simulink model "case4"  (R2024b)
settings: Solver=FixedStepAuto  StartTime=0  StopTime=1  FixedStep=1e-7  RelTol=1e-3
values from neighbouring files (symbols this model uses):
  SG_D_1_D = 0.01056    [IEEE9_case_parameters.m]    (also in case1_parameters.m; case2_parameters.m; case3_parameters.m; case4_parameters.m)
  SG_D_1_EnableSaturation = 0    [IEEE9_case_parameters.m]    (also in case1_parameters.m; case2_parameters.m; case3_parameters.m; case4_parameters.m)
  SG_D_1_f0 = 60    [IEEE9_case_parameters.m]    (also in case1_parameters.m; case2_parameters.m; case3_parameters.m; case4_parameters.m)
  SG_D_1_H = 7.5    [IEEE9_case_parameters.m]    (also in case1_parameters.m; case2_parameters.m; case3_parameters.m; case4_parameters.m)
  SG_D_1_K_A = 20    [IEEE9_case_parameters.m]    (also in case1_parameters.m; case2_parameters.m; case3_parameters.m; case4_parameters.m)
  SG_D_1_K_E = 1.000000e+1    (= 10)    [IEEE9_case_parameters.m]    (also in case1_parameters.m; case2_parameters.m; case3_parameters.m; case4_parameters.m)
  SG_D_1_K_F = 2.363    [IEEE9_case_parameters.m]    (also in case1_parameters.m; case2_parameters.m; case3_parameters.m; case4_parameters.m)
  SG_D_1_K_s = 0.5    [IEEE9_case_parameters.m]    (also in case1_parameters.m = 5; case2_parameters.m = 5; case3_parameters.m = 5; case4_parameters.m = 5)
  SG_D_1_R_a = 0.001088    [IEEE9_case_parameters.m]    (also in case1_parameters.m; case2_parameters.m; case3_parameters.m; case4_parameters.m)
  SG_D_1_S_A = 1    [IEEE9_case_parameters.m]    (also in case1_parameters.m; case2_parameters.m; case3_parameters.m; case4_parameters.m)
  SG_D_1_S_B = 0.103    [IEEE9_case_parameters.m]    (also in case1_parameters.m; case2_parameters.m; case3_parameters.m; case4_parameters.m)
  SG_D_1_S_N = 10.659857    [IEEE9_case_parameters.m]    (also in case1_parameters.m; case2_parameters.m; case3_parameters.m; case4_parameters.m)
  SG_D_1_SpeedPara = 200    [IEEE9_case_parameters.m]    (also in case1_parameters.m; case2_parameters.m; case3_parameters.m; case4_parameters.m)
  SG_D_1_T_0 = 0.720173    [IEEE9_case_parameters.m]    (also in case1_parameters.m = 0.755522; case2_parameters.m = 0.808931; case3_parameters.m = 0.869402; case4_parameters.m = 0.729316)
  SG_D_1_T_1 = 0.3    [IEEE9_case_parameters.m]    (also in case1_parameters.m; case2_parameters.m; case3_parameters.m; case4_parameters.m)
  SG_D_1_T_2 = 0.05    [IEEE9_case_parameters.m]    (also in case1_parameters.m; case2_parameters.m; case3_parameters.m; case4_parameters.m)
  SG_D_1_T_3 = 0.02    [IEEE9_case_parameters.m]    (also in case1_parameters.m; case2_parameters.m; case3_parameters.m; case4_parameters.m)
  SG_D_1_T_4 = 0.005    [IEEE9_case_parameters.m]    (also in case1_parameters.m; case2_parameters.m; case3_parameters.m; case4_parameters.m)
  SG_D_1_T_A = 0.02    [IEEE9_case_parameters.m]    (also in case1_parameters.m; case2_parameters.m; case3_parameters.m; case4_parameters.m)
  SG_D_1_T_dd = 8.000000e+0    (= 8)    [IEEE9_case_parameters.m]    (also in case1_parameters.m; case2_parameters.m; case3_parameters.m; case4_parameters.m)
  SG_D_1_T_ddd = 0.04    [IEEE9_case_parameters.m]    (also in case1_parameters.m; case2_parameters.m; case3_parameters.m; case4_parameters.m)
  SG_D_1_T_E = 0.314    [IEEE9_case_parameters.m]    (also in case1_parameters.m; case2_parameters.m; case3_parameters.m; case4_parameters.m)
  SG_D_1_T_F = 0.35    [IEEE9_case_parameters.m]    (also in case1_parameters.m; case2_parameters.m; case3_parameters.m; case4_parameters.m)
  SG_D_1_T_qd = 0.8    [IEEE9_case_parameters.m]    (also in case1_parameters.m; case2_parameters.m; case3_parameters.m; case4_parameters.m)
  SG_D_1_T_qdd = 0.02    [IEEE9_case_parameters.m]    (also in case1_parameters.m; case2_parameters.m; case3_parameters.m; case4_parameters.m)
  SG_D_1_T_speed = 0.1    [IEEE9_case_parameters.m]    (also in case1_parameters.m = 200; case2_parameters.m = 200; case3_parameters.m = 200; case4_parameters.m = 200)
  SG_D_1_T_w = 0.5    [IEEE9_case_parameters.m]    (also in case1_parameters.m; case2_parameters.m; case3_parameters.m; case4_parameters.m)
  SG_D_1_V_ref = 1.990276    [IEEE9_case_parameters.m]    (also in case1_parameters.m = 2.042296; case2_parameters.m = 2.051388; case3_parameters.m = 2.089584; case4_parameters.m = 2.01845)
  SG_D_1_w_ref = 376.991118    [IEEE9_case_parameters.m]    (also in case1_parameters.m; case2_parameters.m; case3_parameters.m; case4_parameters.m)
  SG_D_1_wb = 6.000000e+1    (= 60)    [IEEE9_case_parameters.m]    (also in case1_parameters.m; case2_parameters.m; case3_parameters.m; case4_parameters.m)
  SG_D_1_x_d = 1.9    [IEEE9_case_parameters.m]    (also in case1_parameters.m; case2_parameters.m; case3_parameters.m; case4_parameters.m)
  SG_D_1_x_dd = 0.302    [IEEE9_case_parameters.m]    (also in case1_parameters.m; case2_parameters.m; case3_parameters.m; case4_parameters.m)
  SG_D_1_x_ddd = 0.204    [IEEE9_case_parameters.m]    (also in case1_parameters.m; case2_parameters.m; case3_parameters.m; case4_parameters.m)
  SG_D_1_x_l = 0.05    [IEEE9_case_parameters.m]    (also in case1_parameters.m; case2_parameters.m; case3_parameters.m; case4_parameters.m)
  SG_D_1_x_q = 1.3    [IEEE9_case_parameters.m]    (also in case1_parameters.m; case2_parameters.m; case3_parameters.m; case4_parameters.m)
  SG_D_1_x_qd = 0.5    [IEEE9_case_parameters.m]    (also in case1_parameters.m; case2_parameters.m; case3_parameters.m; case4_parameters.m)
  SG_D_1_x_qdd = 0.3    [IEEE9_case_parameters.m]    (also in case1_parameters.m; case2_parameters.m; case3_parameters.m; case4_parameters.m)
  SG_D_2_D = 0.02    [IEEE9_case_parameters.m]    (also in case1_parameters.m; case2_parameters.m; case3_parameters.m; case4_parameters.m)
  SG_D_2_EnableSaturation = 0    [IEEE9_case_parameters.m]    (also in case1_parameters.m; case2_parameters.m; case3_parameters.m; case4_parameters.m)
  SG_D_2_f0 = 60    [IEEE9_case_parameters.m]    (also in case1_parameters.m; case2_parameters.m; case3_parameters.m; case4_parameters.m)
  SG_D_2_H = 8.000000e+0    (= 8)    [IEEE9_case_parameters.m]    (also in case1_parameters.m; case2_parameters.m; case3_parameters.m; case4_parameters.m)
  SG_D_2_K_A = 20    [IEEE9_case_parameters.m]    (also in case1_parameters.m; case2_parameters.m; case3_parameters.m; case4_parameters.m)
  SG_D_2_K_E = 1.000000e+1    (= 10)    [IEEE9_case_parameters.m]    (also in case1_parameters.m; case2_parameters.m; case3_parameters.m; case4_parameters.m)
  SG_D_2_K_F = 2.363    [IEEE9_case_parameters.m]    (also in case1_parameters.m; case2_parameters.m; case3_parameters.m; case4_parameters.m)
  SG_D_2_K_s = 0.5    [IEEE9_case_parameters.m]    (also in case1_parameters.m = 4; case2_parameters.m = 4; case3_parameters.m = 4; case4_parameters.m = 4)
  SG_D_2_R_a = 0.001088    [IEEE9_case_parameters.m]    (also in case1_parameters.m; case2_parameters.m; case3_parameters.m; case4_parameters.m)
  SG_D_2_S_A = 1    [IEEE9_case_parameters.m]    (also in case1_parameters.m; case2_parameters.m; case3_parameters.m; case4_parameters.m)
  SG_D_2_S_B = 0.103    [IEEE9_case_parameters.m]    (also in case1_parameters.m; case2_parameters.m; case3_parameters.m; case4_parameters.m)
  SG_D_2_S_N = 10.659857    [IEEE9_case_parameters.m]    (also in case1_parameters.m; case2_parameters.m; case3_parameters.m; case4_parameters.m)
  SG_D_2_SpeedPara = 200    [IEEE9_case_parameters.m]    (also in case1_parameters.m; case2_parameters.m; case3_parameters.m; case4_parameters.m)
  SG_D_2_T_0 = 1.632913    [IEEE9_case_parameters.m]    (also in case1_parameters.m = 1.632925; case2_parameters.m = 1.632915; case3_parameters.m = 1.632914; case4_parameters.m = 1.632927)
  SG_D_2_T_1 = 0.2    [IEEE9_case_parameters.m]    (also in case1_parameters.m; case2_parameters.m; case3_parameters.m; case4_parameters.m)
  SG_D_2_T_2 = 0.05    [IEEE9_case_parameters.m]    (also in case1_parameters.m; case2_parameters.m; case3_parameters.m; case4_parameters.m)
  SG_D_2_T_3 = 0.02    [IEEE9_case_parameters.m]    (also in case1_parameters.m; case2_parameters.m; case3_parameters.m; case4_parameters.m)
  SG_D_2_T_4 = 0.005    [IEEE9_case_parameters.m]    (also in case1_parameters.m; case2_parameters.m; case3_parameters.m; case4_parameters.m)
  SG_D_2_T_A = 0.02    [IEEE9_case_parameters.m]    (also in case1_parameters.m; case2_parameters.m; case3_parameters.m; case4_parameters.m)
  SG_D_2_T_dd = 7.9    [IEEE9_case_parameters.m]    (also in case1_parameters.m; case2_parameters.m; case3_parameters.m; case4_parameters.m)
  SG_D_2_T_ddd = 0.04    [IEEE9_case_parameters.m]    (also in case1_parameters.m; case2_parameters.m; case3_parameters.m; case4_parameters.m)
  SG_D_2_T_E = 0.314    [IEEE9_case_parameters.m]    (also in case1_parameters.m; case2_parameters.m; case3_parameters.m; case4_parameters.m)
  SG_D_2_T_F = 0.35    [IEEE9_case_parameters.m]    (also in case1_parameters.m; case2_parameters.m; case3_parameters.m; case4_parameters.m)
  SG_D_2_T_qd = 0.8    [IEEE9_case_parameters.m]    (also in case1_parameters.m; case2_parameters.m; case3_parameters.m; case4_parameters.m)
  SG_D_2_T_qdd = 0.015    [IEEE9_case_parameters.m]    (also in case1_parameters.m; case2_parameters.m; case3_parameters.m; case4_parameters.m)
  SG_D_2_T_speed = 0.1    [IEEE9_case_parameters.m]    (also in case1_parameters.m = 150; case2_parameters.m = 150; case3_parameters.m = 150; case4_parameters.m = 150)
  SG_D_2_T_w = 0.35    [IEEE9_case_parameters.m]    (also in case1_parameters.m; case2_parameters.m; case3_parameters.m; case4_parameters.m)
  SG_D_2_V_ref = 2.58547    [IEEE9_case_parameters.m]    (also in case1_parameters.m = 2.597896; case2_parameters.m = 2.587136; case3_parameters.m = 2.586042; case4_parameters.m = 2.599679)
  SG_D_2_w_ref = 376.991118    [IEEE9_case_parameters.m]    (also in case1_parameters.m; case2_parameters.m; case3_parameters.m; case4_parameters.m)
  SG_D_2_wb = 6.000000e+1    (= 60)    [IEEE9_case_parameters.m]    (also in case1_parameters.m; case2_parameters.m; case3_parameters.m; case4_parameters.m)
  SG_D_2_x_d = 1.8    [IEEE9_case_parameters.m]    (also in case1_parameters.m; case2_parameters.m; case3_parameters.m; case4_parameters.m)
  SG_D_2_x_dd = 0.302    [IEEE9_case_parameters.m]    (also in case1_parameters.m; case2_parameters.m; case3_parameters.m; case4_parameters.m)
  SG_D_2_x_ddd = 0.204    [IEEE9_case_parameters.m]    (also in case1_parameters.m; case2_parameters.m; case3_parameters.m; case4_parameters.m)
  SG_D_2_x_l = 0.05    [IEEE9_case_parameters.m]    (also in case1_parameters.m; case2_parameters.m; case3_parameters.m; case4_parameters.m)
  SG_D_2_x_q = 1.25    [IEEE9_case_parameters.m]    (also in case1_parameters.m; case2_parameters.m; case3_parameters.m; case4_parameters.m)
  SG_D_2_x_qd = 0.5    [IEEE9_case_parameters.m]    (also in case1_parameters.m; case2_parameters.m; case3_parameters.m; case4_parameters.m)
  SG_D_2_x_qdd = 0.3    [IEEE9_case_parameters.m]    (also in case1_parameters.m; case2_parameters.m; case3_parameters.m; case4_parameters.m)
  SG_D_3_D = 0.02    [IEEE9_case_parameters.m]    (also in case1_parameters.m; case2_parameters.m; case3_parameters.m; case4_parameters.m)
  SG_D_3_EnableSaturation = 0    [IEEE9_case_parameters.m]    (also in case1_parameters.m; case2_parameters.m; case3_parameters.m; case4_parameters.m)
  SG_D_3_f0 = 60    [IEEE9_case_parameters.m]    (also in case1_parameters.m; case2_parameters.m; case3_parameters.m; case4_parameters.m)
  SG_D_3_H = 7.7    [IEEE9_case_parameters.m]    (also in case1_parameters.m; case2_parameters.m; case3_parameters.m; case4_parameters.m)
  SG_D_3_K_A = 20    [IEEE9_case_parameters.m]    (also in case1_parameters.m; case2_parameters.m; case3_parameters.m; case4_parameters.m)
  SG_D_3_K_E = 1.000000e+1    (= 10)    [IEEE9_case_parameters.m]    (also in case1_parameters.m; case2_parameters.m; case3_parameters.m; case4_parameters.m)
  SG_D_3_K_F = 2.363    [IEEE9_case_parameters.m]    (also in case1_parameters.m; case2_parameters.m; case3_parameters.m; case4_parameters.m)
  SG_D_3_K_s = 0.2    [IEEE9_case_parameters.m]    (also in case1_parameters.m = 2; case2_parameters.m = 2; case3_parameters.m = 2; case4_parameters.m = 2)
  SG_D_3_R_a = 0.001088    [IEEE9_case_parameters.m]    (also in case1_parameters.m; case2_parameters.m; case3_parameters.m; case4_parameters.m)
  SG_D_3_S_A = 1    [IEEE9_case_parameters.m]    (also in case1_parameters.m; case2_parameters.m; case3_parameters.m; case4_parameters.m)
  SG_D_3_S_B = 0.103    [IEEE9_case_parameters.m]    (also in case1_parameters.m; case2_parameters.m; case3_parameters.m; case4_parameters.m)
  SG_D_3_S_N = 10.659857    [IEEE9_case_parameters.m]    (also in case1_parameters.m; case2_parameters.m; case3_parameters.m; case4_parameters.m)
  SG_D_3_SpeedPara = 200    [IEEE9_case_parameters.m]    (also in case1_parameters.m; case2_parameters.m; case3_parameters.m; case4_parameters.m)
  SG_D_3_T_0 = 0.850788    [IEEE9_case_parameters.m]    (also in case1_parameters.m = 0.850786; case2_parameters.m = 0.850787; case3_parameters.m; case4_parameters.m = 0.850786)
  SG_D_3_T_1 = 0.2    [IEEE9_case_parameters.m]    (also in case1_parameters.m; case2_parameters.m; case3_parameters.m; case4_parameters.m)
  SG_D_3_T_2 = 0.05    [IEEE9_case_parameters.m]    (also in case1_parameters.m; case2_parameters.m; case3_parameters.m; case4_parameters.m)
  SG_D_3_T_3 = 0.02    [IEEE9_case_parameters.m]    (also in case1_parameters.m; case2_parameters.m; case3_parameters.m; case4_parameters.m)
  SG_D_3_T_4 = 0.005    [IEEE9_case_parameters.m]    (also in case1_parameters.m; case2_parameters.m; case3_parameters.m; case4_parameters.m)
  SG_D_3_T_A = 0.02    [IEEE9_case_parameters.m]    (also in case1_parameters.m; case2_parameters.m; case3_parameters.m; case4_parameters.m)
  SG_D_3_T_dd = 8.1    [IEEE9_case_parameters.m]    (also in case1_parameters.m; case2_parameters.m; case3_parameters.m; case4_parameters.m)
  SG_D_3_T_ddd = 0.04    [IEEE9_case_parameters.m]    (also in case1_parameters.m; case2_parameters.m; case3_parameters.m; case4_parameters.m)
  SG_D_3_T_E = 0.314    [IEEE9_case_parameters.m]    (also in case1_parameters.m; case2_parameters.m; case3_parameters.m; case4_parameters.m)
  SG_D_3_T_F = 0.35    [IEEE9_case_parameters.m]    (also in case1_parameters.m; case2_parameters.m; case3_parameters.m; case4_parameters.m)
  SG_D_3_T_qd = 0.8    [IEEE9_case_parameters.m]    (also in case1_parameters.m; case2_parameters.m; case3_parameters.m; case4_parameters.m)
  SG_D_3_T_qdd = 0.015    [IEEE9_case_parameters.m]    (also in case1_parameters.m; case2_parameters.m; case3_parameters.m; case4_parameters.m)
  SG_D_3_T_speed = 0.1    [IEEE9_case_parameters.m]    (also in case1_parameters.m = 180; case2_parameters.m = 180; case3_parameters.m = 180; case4_parameters.m = 180)
  SG_D_3_T_w = 0.4    [IEEE9_case_parameters.m]    (also in case1_parameters.m; case2_parameters.m; case3_parameters.m; case4_parameters.m)
  SG_D_3_V_ref = 1.892727    [IEEE9_case_parameters.m]    (also in case1_parameters.m = 1.906439; case2_parameters.m = 1.895535; case3_parameters.m = 1.892105; case4_parameters.m = 1.906598)
  SG_D_3_w_ref = 376.991118    [IEEE9_case_parameters.m]    (also in case1_parameters.m; case2_parameters.m; case3_parameters.m; case4_parameters.m)
  SG_D_3_wb = 6.000000e+1    (= 60)    [IEEE9_case_parameters.m]    (also in case1_parameters.m; case2_parameters.m; case3_parameters.m; case4_parameters.m)
  SG_D_3_x_d = 1.85    [IEEE9_case_parameters.m]    (also in case1_parameters.m; case2_parameters.m; case3_parameters.m; case4_parameters.m)
  SG_D_3_x_dd = 0.302    [IEEE9_case_parameters.m]    (also in case1_parameters.m; case2_parameters.m; case3_parameters.m; case4_parameters.m)
  SG_D_3_x_ddd = 0.204    [IEEE9_case_parameters.m]    (also in case1_parameters.m; case2_parameters.m; case3_parameters.m; case4_parameters.m)
  SG_D_3_x_l = 0.05    [IEEE9_case_parameters.m]    (also in case1_parameters.m; case2_parameters.m; case3_parameters.m; case4_parameters.m)
  SG_D_3_x_q = 1.2    [IEEE9_case_parameters.m]    (also in case1_parameters.m; case2_parameters.m; case3_parameters.m; case4_parameters.m)
  SG_D_3_x_qd = 0.5    [IEEE9_case_parameters.m]    (also in case1_parameters.m; case2_parameters.m; case3_parameters.m; case4_parameters.m)
  SG_D_3_x_qdd = 0.3    [IEEE9_case_parameters.m]    (also in case1_parameters.m; case2_parameters.m; case3_parameters.m; case4_parameters.m)
(part 3 of 12)

== system case4/AC_1/d_id_load_7_block ==
  note: d_id_load_7 in case4
      | $376.991118430775\,\mathrm{iq}_{\mathrm{load},7}-1028.49421693228\,\mathrm{id}_{\mathrm{load},7}+1212.41742610852\,\mathrm{vd}_{\mathrm{bus},7}$
      | Automatically generated on 2025-10-31 19:07:38 .
  State_id_load_7_751d5 : Inport
  State_iq_load_7_8050b : Inport  Port=2
  State_vd_bus_7_9625b : Inport  Port=3
  Add_933b8 : Sum
  Add_aa192 : Sum
  Constant_-1028.49421693228_0e231 : Constant  Value=-1028.49421693228
  Constant_1212.41742610852_091cd : Constant  Value=1212.41742610852
  Constant_376.991118430775_fc973 : Constant  Value=376.991118430775
  Product_071bf : Product
  Product_29fc2 : Product
  Product_cece1 : Product
  Blockout_d_id_load_7_d2cec : Outport
  wires:
  Constant_-1028.49421693228_0e231/1 -> Product_cece1/1
  Product_29fc2/1 -> Add_aa192/2
  State_id_load_7_751d5/1 -> Product_cece1/2
  Constant_376.991118430775_fc973/1 -> Product_29fc2/1
  Product_cece1/1 -> Add_aa192/1
  State_iq_load_7_8050b/1 -> Product_29fc2/2
  Constant_1212.41742610852_091cd/1 -> Product_071bf/1
  State_vd_bus_7_9625b/1 -> Product_071bf/2
  Add_aa192/1 -> Add_933b8/1
  Product_071bf/1 -> Add_933b8/2
  Add_933b8/1 -> Blockout_d_id_load_7_d2cec/1

== system case4/AC_1/d_id_load_9_block ==
  note: d_id_load_9 in case4
      | $376.991118430775\,\mathrm{iq}_{\mathrm{load},9}-899.932439784723\,\mathrm{id}_{\mathrm{load},9}+1462.33884976487\,\mathrm{vd}_{\mathrm{bus},9}$
      | Automatically generated on 2025-10-31 19:07:40 .
  State_id_load_9_aba5e : Inport
  State_iq_load_9_24674 : Inport  Port=2
  State_vd_bus_9_72280 : Inport  Port=3
  Add_3686a : Sum
  Add_ba33a : Sum
  Constant_-899.932439784723_46537 : Constant  Value=-899.932439784723
  Constant_1462.33884976487_f6216 : Constant  Value=1462.33884976487
  Constant_376.991118430775_89578 : Constant  Value=376.991118430775
  Product_3b7f2 : Product
  Product_84f3a : Product
  Product_e126b : Product
  Blockout_d_id_load_9_04629 : Outport
  wires:
  Constant_-899.932439784723_46537/1 -> Product_e126b/1
  Product_84f3a/1 -> Add_ba33a/2
  State_id_load_9_aba5e/1 -> Product_e126b/2
  Constant_376.991118430775_89578/1 -> Product_84f3a/1
  Product_e126b/1 -> Add_ba33a/1
  State_iq_load_9_24674/1 -> Product_84f3a/2
  Constant_1462.33884976487_f6216/1 -> Product_3b7f2/1
  State_vd_bus_9_72280/1 -> Product_3b7f2/2
  Add_ba33a/1 -> Add_3686a/1
  Product_3b7f2/1 -> Add_3686a/2
  Add_3686a/1 -> Blockout_d_id_load_9_04629/1

== system case4/AC_1/d_iq_line_1_4_block ==
  note: d_iq_line_1_4 in case4
      | $6254.53843232971\,\mathrm{vq}_{\mathrm{bus},1}-376.991118430775\,\mathrm{id}_{\mathrm{line},1,4}-6254.53843232971\,\mathrm{vq}_{\mathrm{bus},4}$
      | Automatically generated on 2025-10-31 19:07:43 .
  State_id_line_1_4_0dfc6 : Inport
  State_vq_bus_1_71810 : Inport  Port=2
  State_vq_bus_4_452a3 : Inport  Port=3
  Add_ee138 : Sum
  Constant_-376.991118430775_59d54 : Constant  Value=-376.991118430775
  Constant_6254.53843232971_48952 : Constant  Value=6254.53843232971
  Constant_6254.53843232971_c9a73 : Constant  Value=6254.53843232971
  Product_0f1ea : Product
  Product_db189 : Product
  Product_f7492 : Product
  Subtract_9dc84 : Sum  Inputs=+-
  Blockout_d_iq_line_1_4_15027 : Outport
  wires:
  Constant_-376.991118430775_59d54/1 -> Product_0f1ea/1
  Product_db189/1 -> Add_ee138/2
  State_id_line_1_4_0dfc6/1 -> Product_0f1ea/2
  Constant_6254.53843232971_48952/1 -> Product_db189/1
  Product_0f1ea/1 -> Add_ee138/1
  Subtract_9dc84/1 -> Blockout_d_iq_line_1_4_15027/1
  State_vq_bus_1_71810/1 -> Product_db189/2
  Constant_6254.53843232971_c9a73/1 -> Product_f7492/1
  State_vq_bus_4_452a3/1 -> Product_f7492/2
  Add_ee138/1 -> Subtract_9dc84/1
  Product_f7492/1 -> Subtract_9dc84/2

== system case4/AC_1/d_iq_line_3_6_block ==
  note: d_iq_line_3_6 in case4
      | $6147.80569457664\,\mathrm{vq}_{\mathrm{bus},3}-376.991118430775\,\mathrm{id}_{\mathrm{line},3,6}-6147.80569457664\,\mathrm{vq}_{\mathrm{bus},6}$
      | Automatically generated on 2025-10-31 19:07:50 .
  State_id_line_3_6_92370 : Inport
  State_vq_bus_3_67a70 : Inport  Port=2
  State_vq_bus_6_0d319 : Inport  Port=3
  Add_54a1e : Sum
  Constant_-376.991118430775_80b53 : Constant  Value=-376.991118430775
  Constant_6147.80569457664_b1c13 : Constant  Value=6147.80569457664
  Constant_6147.80569457664_bf027 : Constant  Value=6147.80569457664
  Product_3d920 : Product
  Product_52216 : Product
  Product_cc0ed : Product
  Subtract_6c621 : Sum  Inputs=+-
  Blockout_d_iq_line_3_6_89b36 : Outport
  wires:
  Constant_-376.991118430775_80b53/1 -> Product_3d920/1
  Product_cc0ed/1 -> Add_54a1e/2
  State_id_line_3_6_92370/1 -> Product_3d920/2
  Constant_6147.80569457664_bf027/1 -> Product_cc0ed/1
  Product_3d920/1 -> Add_54a1e/1
  State_vq_bus_3_67a70/1 -> Product_cc0ed/2
  Constant_6147.80569457664_b1c13/1 -> Product_52216/1
  State_vq_bus_6_0d319/1 -> Product_52216/2
  Add_54a1e/1 -> Subtract_6c621/1
  Product_52216/1 -> Subtract_6c621/2
  Subtract_6c621/1 -> Blockout_d_iq_line_3_6_89b36/1

== system case4/AC_1/d_iq_line_4_5_block ==
  note: d_iq_line_4_5 in case4
      | $3915.88493154556\,\mathrm{vq}_{\mathrm{bus},4}-66.2754255159152\,\mathrm{iq}_{\mathrm{line},4,5}-376.991118430775\,\mathrm{id}_{\mathrm{line},4,5}-3915.88493154556\,\mathrm{vq}_{\mathrm{bus},5}$
      | Automatically generated on 2025-10-31 19:07:46 .
  State_id_line_4_5_4cdcf : Inport
  State_iq_line_4_5_de839 : Inport  Port=2
  State_vq_bus_4_cf608 : Inport  Port=3
  State_vq_bus_5_37393 : Inport  Port=4
  Add_02ce2 : Sum
  Constant_-376.991118430775_da52a : Constant  Value=-376.991118430775
  Constant_3915.88493154556_78018 : Constant  Value=3915.88493154556
  Constant_3915.88493154556_aaaab : Constant  Value=3915.88493154556
  Constant_66.2754255159152_51cb1 : Constant  Value=66.2754255159152
  Product_0924f : Product
  Product_3af8c : Product
  Product_8200f : Product
  Product_f63e0 : Product
  Subtract_81fb3 : Sum  Inputs=+-
  Subtract_ff1e7 : Sum  Inputs=+-
  Blockout_d_iq_line_4_5_800d2 : Outport
  wires:
  Constant_-376.991118430775_da52a/1 -> Product_0924f/1
  Constant_66.2754255159152_51cb1/1 -> Product_3af8c/1
  State_id_line_4_5_4cdcf/1 -> Product_0924f/2
  State_iq_line_4_5_de839/1 -> Product_3af8c/2
  Product_0924f/1 -> Subtract_ff1e7/1
  Constant_3915.88493154556_aaaab/1 -> Product_f63e0/1
  Product_3af8c/1 -> Subtract_ff1e7/2
  State_vq_bus_4_cf608/1 -> Product_f63e0/2
  Subtract_ff1e7/1 -> Add_02ce2/1
  Product_f63e0/1 -> Add_02ce2/2
  Constant_3915.88493154556_78018/1 -> Product_8200f/1
  State_vq_bus_5_37393/1 -> Product_8200f/2
  Add_02ce2/1 -> Subtract_81fb3/1
  Product_8200f/1 -> Subtract_81fb3/2
  Subtract_81fb3/1 -> Blockout_d_iq_line_4_5_800d2/1

== system case4/AC_1/d_iq_line_5_6_block ==
  note: d_iq_line_5_6 in case4
      | $2119.18478648348\,\mathrm{vq}_{\mathrm{bus},5}-82.282431401766\,\mathrm{iq}_{\mathrm{line},5,6}-376.991118430775\,\mathrm{id}_{\mathrm{line},5,6}-2119.18478648348\,\mathrm{vq}_{\mathrm{bus},6}$
      | Automatically generated on 2025-10-31 19:07:48 .
  State_id_line_5_6_cde43 : Inport
  State_iq_line_5_6_96bf5 : Inport  Port=2
  State_vq_bus_5_29364 : Inport  Port=3
  State_vq_bus_6_3bcbb : Inport  Port=4
  Add_ff1d7 : Sum
  Constant_-376.991118430775_3d086 : Constant  Value=-376.991118430775
  Constant_2119.18478648348_0c142 : Constant  Value=2119.18478648348
  Constant_2119.18478648348_361ec : Constant  Value=2119.18478648348
  Constant_82.282431401766_06879 : Constant  Value=82.282431401766
  Product_172a5 : Product
  Product_23624 : Product
  Product_478ae : Product
  Product_dfd52 : Product
  Subtract_2b357 : Sum  Inputs=+-
  Subtract_dd82d : Sum  Inputs=+-
  Blockout_d_iq_line_5_6_b33bc : Outport
  wires:
  Constant_-376.991118430775_3d086/1 -> Product_23624/1
  Constant_82.282431401766_06879/1 -> Product_172a5/1
  Subtract_dd82d/1 -> Blockout_d_iq_line_5_6_b33bc/1
  State_id_line_5_6_cde43/1 -> Product_23624/2
  State_iq_line_5_6_96bf5/1 -> Product_172a5/2
  Product_23624/1 -> Subtract_2b357/1
  Constant_2119.18478648348_361ec/1 -> Product_dfd52/1
  Product_172a5/1 -> Subtract_2b357/2
  Product_478ae/1 -> Subtract_dd82d/2
  State_vq_bus_5_29364/1 -> Product_dfd52/2
  Subtract_2b357/1 -> Add_ff1d7/1
  Product_dfd52/1 -> Add_ff1d7/2
  Constant_2119.18478648348_0c142/1 -> Product_478ae/1
  State_vq_bus_6_3bcbb/1 -> Product_478ae/2
  Add_ff1d7/1 -> Subtract_dd82d/1

== system case4/AC_1/d_iq_line_6_7_block ==
  note: d_iq_line_6_7 in case4
      | $3574.02196133126\,\mathrm{vq}_{\mathrm{bus},6}-42.3426329685014\,\mathrm{iq}_{\mathrm{line},6,7}-376.991118430775\,\mathrm{id}_{\mathrm{line},6,7}-3574.02196133126\,\mathrm{vq}_{\mathrm{bus},7}$
      | Automatically generated on 2025-10-31 19:07:53 .
  State_id_line_6_7_c49e4 : Inport
  State_iq_line_6_7_f03d7 : Inport  Port=2
  State_vq_bus_6_ae467 : Inport  Port=3
  State_vq_bus_7_ffa00 : Inport  Port=4
  Add_7372f : Sum
  Constant_-376.991118430775_18e8e : Constant  Value=-376.991118430775
  Constant_3574.02196133126_34ec0 : Constant  Value=3574.02196133126
  Constant_3574.02196133126_bf393 : Constant  Value=3574.02196133126
  Constant_42.3426329685014_20b8e : Constant  Value=42.3426329685014
  Product_058d9 : Product
  Product_22266 : Product
  Product_2a12e : Product
  Product_68ad9 : Product
  Subtract_1c7db : Sum  Inputs=+-
  Subtract_97b8c : Sum  Inputs=+-
  Blockout_d_iq_line_6_7_229ae : Outport
  wires:
  Constant_-376.991118430775_18e8e/1 -> Product_22266/1
  Constant_42.3426329685014_20b8e/1 -> Product_058d9/1
  State_id_line_6_7_c49e4/1 -> Product_22266/2
  State_iq_line_6_7_f03d7/1 -> Product_058d9/2
  Product_22266/1 -> Subtract_97b8c/1
  Constant_3574.02196133126_34ec0/1 -> Product_68ad9/1
  Product_058d9/1 -> Subtract_97b8c/2
  State_vq_bus_6_ae467/1 -> Product_68ad9/2
  Subtract_97b8c/1 -> Add_7372f/1
  Product_68ad9/1 -> Add_7372f/2
  Constant_3574.02196133126_bf393/1 -> Product_2a12e/1
  State_vq_bus_7_ffa00/1 -> Product_2a12e/2
  Add_7372f/1 -> Subtract_1c7db/1
  Product_2a12e/1 -> Subtract_1c7db/2
  Subtract_1c7db/1 -> Blockout_d_iq_line_6_7_229ae/1

== system case4/AC_1/d_iq_line_7_8_block ==
  note: d_iq_line_7_8 in case4
      | $5003.63074586377\,\mathrm{vq}_{\mathrm{bus},7}-42.3426329685014\,\mathrm{iq}_{\mathrm{line},7,8}-376.991118430775\,\mathrm{id}_{\mathrm{line},7,8}-5003.63074586377\,\mathrm{vq}_{\mathrm{bus},8}$
      | Automatically generated on 2025-10-31 19:07:55 .
  State_id_line_7_8_e42a6 : Inport
  State_iq_line_7_8_485ac : Inport  Port=2
  State_vq_bus_7_d0e8e : Inport  Port=3
  State_vq_bus_8_897ad : Inport  Port=4
  Add_4a3fb : Sum
  Constant_-376.991118430775_bb795 : Constant  Value=-376.991118430775
  Constant_42.3426329685014_aae9d : Constant  Value=42.3426329685014
  Constant_5003.63074586377_78c4a : Constant  Value=5003.63074586377
  Constant_5003.63074586377_d7046 : Constant  Value=5003.63074586377
  Product_0b0c0 : Product
  Product_32409 : Product
  Product_ba38c : Product
  Product_fe0ff : Product
  Subtract_8b7af : Sum  Inputs=+-
  Subtract_dc337 : Sum  Inputs=+-
  Blockout_d_iq_line_7_8_fee52 : Outport
  wires:
  Constant_-376.991118430775_bb795/1 -> Product_0b0c0/1
  Constant_42.3426329685014_aae9d/1 -> Product_ba38c/1
  State_id_line_7_8_e42a6/1 -> Product_0b0c0/2
  State_iq_line_7_8_485ac/1 -> Product_ba38c/2
  Product_0b0c0/1 -> Subtract_dc337/1
  Constant_5003.63074586377_d7046/1 -> Product_32409/1
  Product_ba38c/1 -> Subtract_dc337/2
  State_vq_bus_7_d0e8e/1 -> Product_32409/2
  Subtract_dc337/1 -> Add_4a3fb/1
  Product_32409/1 -> Add_4a3fb/2
  Constant_5003.63074586377_78c4a/1 -> Product_fe0ff/1
  State_vq_bus_8_897ad/1 -> Product_fe0ff/2
  Add_4a3fb/1 -> Subtract_8b7af/1
  Product_fe0ff/1 -> Subtract_8b7af/2
  Subtract_8b7af/1 -> Blockout_d_iq_line_7_8_fee52/1

== system case4/AC_1/d_iq_line_8_2_block ==
  note: d_iq_line_8_2 in case4
      | $5764.18261923506\,\mathrm{vq}_{\mathrm{bus},8}-5764.18261923506\,\mathrm{vq}_{\mathrm{bus},2}-376.991118430775\,\mathrm{id}_{\mathrm{line},8,2}$
      | Automatically generated on 2025-10-31 19:07:57 .
  State_id_line_8_2_1a66c : Inport
  State_vq_bus_2_c1e81 : Inport  Port=2
  State_vq_bus_8_7ea40 : Inport  Port=3
  Add_1f3ad : Sum
  Constant_-376.991118430775_408e8 : Constant  Value=-376.991118430775
  Constant_5764.18261923506_3a7a6 : Constant  Value=5764.18261923506
  Constant_5764.18261923506_b2b7d : Constant  Value=5764.18261923506
  Product_077a7 : Product
  Product_6a578 : Product
  Product_76284 : Product
  Subtract_39bfc : Sum  Inputs=+-
  Blockout_d_iq_line_8_2_851f9 : Outport
  wires:
  Constant_-376.991118430775_408e8/1 -> Product_077a7/1
  Product_76284/1 -> Subtract_39bfc/2
  State_id_line_8_2_1a66c/1 -> Product_077a7/2
  Constant_5764.18261923506_b2b7d/1 -> Product_76284/1
  Product_077a7/1 -> Subtract_39bfc/1
  State_vq_bus_2_c1e81/1 -> Product_76284/2
  Constant_5764.18261923506_3a7a6/1 -> Product_6a578/1
  State_vq_bus_8_7ea40/1 -> Product_6a578/2
  Subtract_39bfc/1 -> Add_1f3ad/1
  Product_6a578/1 -> Add_1f3ad/2
  Add_1f3ad/1 -> Blockout_d_iq_line_8_2_851f9/1

== system case4/AC_1/d_iq_line_8_9_block ==
  note: d_iq_line_8_9 in case4
      | $2237.64853231175\,\mathrm{vq}_{\mathrm{bus},8}-71.2878526557744\,\mathrm{iq}_{\mathrm{line},8,9}-376.991118430775\,\mathrm{id}_{\mathrm{line},8,9}-2237.64853231175\,\mathrm{vq}_{\mathrm{bus},9}$
      | Automatically generated on 2025-10-31 19:08:00 .
  State_id_line_8_9_6dd72 : Inport
  State_iq_line_8_9_3cc7e : Inport  Port=2
  State_vq_bus_8_6d34c : Inport  Port=3
  State_vq_bus_9_b3300 : Inport  Port=4
  Add_922f7 : Sum
  Constant_-376.991118430775_b157b : Constant  Value=-376.991118430775
  Constant_2237.64853231175_69d50 : Constant  Value=2237.64853231175
  Constant_2237.64853231175_97245 : Constant  Value=2237.64853231175
  Constant_71.2878526557744_839ee : Constant  Value=71.2878526557744
  Product_43596 : Product
  Product_5606c : Product
  Product_e4a79 : Product
  Product_f42fb : Product
  Subtract_ac73f : Sum  Inputs=+-
  Subtract_f2c5f : Sum  Inputs=+-
  Blockout_d_iq_line_8_9_05116 : Outport
  wires:
  Constant_-376.991118430775_b157b/1 -> Product_e4a79/1
  Constant_71.2878526557744_839ee/1 -> Product_43596/1
  State_id_line_8_9_6dd72/1 -> Product_e4a79/2
  State_iq_line_8_9_3cc7e/1 -> Product_43596/2
  Product_e4a79/1 -> Subtract_f2c5f/1
  Constant_2237.64853231175_97245/1 -> Product_5606c/1
  Product_43596/1 -> Subtract_f2c5f/2
  State_vq_bus_8_6d34c/1 -> Product_5606c/2
  Subtract_f2c5f/1 -> Add_922f7/1
  Product_5606c/1 -> Add_922f7/2
  Constant_2237.64853231175_69d50/1 -> Product_f42fb/1
  Add_922f7/1 -> Subtract_ac73f/1
  State_vq_bus_9_b3300/1 -> Product_f42fb/2
  Product_f42fb/1 -> Subtract_ac73f/2
  Subtract_ac73f/1 -> Blockout_d_iq_line_8_9_05116/1

== system case4/AC_1/d_iq_line_9_4_block ==
  note: d_iq_line_9_4 in case4
      | $4238.36957296695\,\mathrm{vq}_{\mathrm{bus},9}-42.1961186675723\,\mathrm{iq}_{\mathrm{line},9,4}-4238.36957296695\,\mathrm{vq}_{\mathrm{bus},4}-376.991118430775\,\mathrm{id}_{\mathrm{line},9,4}$
      | Automatically generated on 2025-10-31 19:08:02 .
  State_id_line_9_4_f5685 : Inport
  State_iq_line_9_4_10a5e : Inport  Port=2
  State_vq_bus_4_9407e : Inport  Port=3
  State_vq_bus_9_e7522 : Inport  Port=4
  Add_c1361 : Sum
  Constant_-376.991118430775_3c590 : Constant  Value=-376.991118430775
  Constant_42.1961186675723_96edb : Constant  Value=42.1961186675723
  Constant_4238.36957296695_0a917 : Constant  Value=4238.36957296695
  Constant_4238.36957296695_3c0ee : Constant  Value=4238.36957296695
  Product_91c1a : Product
  Product_a6017 : Product
  Product_f9bb3 : Product
  Product_fcd36 : Product
  Subtract_662d3 : Sum  Inputs=+-
  Subtract_8573e : Sum  Inputs=+-
  Blockout_d_iq_line_9_4_8eaf6 : Outport
  wires:
  Constant_-376.991118430775_3c590/1 -> Product_fcd36/1
  Constant_42.1961186675723_96edb/1 -> Product_a6017/1
  State_id_line_9_4_f5685/1 -> Product_fcd36/2
  State_iq_line_9_4_10a5e/1 -> Product_a6017/2
  Product_fcd36/1 -> Subtract_662d3/1
  Constant_4238.36957296695_3c0ee/1 -> Product_f9bb3/1
  Product_a6017/1 -> Subtract_662d3/2
  State_vq_bus_4_9407e/1 -> Product_f9bb3/2
  Subtract_662d3/1 -> Subtract_8573e/1
  Product_f9bb3/1 -> Subtract_8573e/2
  Constant_4238.36957296695_0a917/1 -> Product_91c1a/1
  Add_c1361/1 -> Blockout_d_iq_line_9_4_8eaf6/1
  State_vq_bus_9_e7522/1 -> Product_91c1a/2
  Subtract_8573e/1 -> Add_c1361/1
  Product_91c1a/1 -> Add_c1361/2

== system case4/AC_1/d_iq_load_5_block ==
  note: d_iq_load_5 in case4
      | $1157.47551177004\,\mathrm{vq}_{\mathrm{bus},5}-1079.91892759499\,\mathrm{iq}_{\mathrm{load},5}-376.991118430775\,\mathrm{id}_{\mathrm{load},5}$
      | Automatically generated on 2025-10-31 19:07:37 .
  State_id_load_5_f6e5b : Inport
  State_iq_load_5_28b96 : Inport  Port=2
  State_vq_bus_5_534fe : Inport  Port=3
  Add_5e245 : Sum
  Constant_-376.991118430775_05236 : Constant  Value=-376.991118430775
  Constant_1079.91892759499_2fc55 : Constant  Value=1079.91892759499
  Constant_1157.47551177004_9aaa0 : Constant  Value=1157.47551177004
  Product_767c6 : Product
  Product_7fed4 : Product
  Product_ac8e7 : Product
  Subtract_e17a7 : Sum  Inputs=+-
  Blockout_d_iq_load_5_f01ab : Outport
  wires:
  Constant_-376.991118430775_05236/1 -> Product_767c6/1
  Product_ac8e7/1 -> Subtract_e17a7/2
  State_id_load_5_f6e5b/1 -> Product_767c6/2
  Constant_1079.91892759499_2fc55/1 -> Product_ac8e7/1
  Product_767c6/1 -> Subtract_e17a7/1
  State_iq_load_5_28b96/1 -> Product_ac8e7/2
  Constant_1157.47551177004_9aaa0/1 -> Product_7fed4/1
  State_vq_bus_5_534fe/1 -> Product_7fed4/2
  Subtract_e17a7/1 -> Add_5e245/1
  Product_7fed4/1 -> Add_5e245/2
  Add_5e245/1 -> Blockout_d_iq_load_5_f01ab/1

== system case4/AC_1/d_iq_load_7_block ==
  note: d_iq_load_7 in case4
      | $1212.41742610852\,\mathrm{vq}_{\mathrm{bus},7}-1028.49421693228\,\mathrm{iq}_{\mathrm{load},7}-376.991118430775\,\mathrm{id}_{\mathrm{load},7}$
      | Automatically generated on 2025-10-31 19:07:39 .
  State_id_load_7_6612a : Inport
  State_iq_load_7_2144d : Inport  Port=2
  State_vq_bus_7_6865b : Inport  Port=3
  Add_32508 : Sum
  Constant_-376.991118430775_47c14 : Constant  Value=-376.991118430775
  Constant_1028.49421693228_de725 : Constant  Value=1028.49421693228
  Constant_1212.41742610852_0f8ee : Constant  Value=1212.41742610852
  Product_108d3 : Product
  Product_7e168 : Product
  Product_b1a08 : Product
  Subtract_4f174 : Sum  Inputs=+-
  Blockout_d_iq_load_7_52844 : Outport
  wires:
  Constant_-376.991118430775_47c14/1 -> Product_b1a08/1
  Product_108d3/1 -> Subtract_4f174/2
  State_id_load_7_6612a/1 -> Product_b1a08/2
  Constant_1028.49421693228_de725/1 -> Product_108d3/1
  Product_b1a08/1 -> Subtract_4f174/1
  State_iq_load_7_2144d/1 -> Product_108d3/2
  Constant_1212.41742610852_0f8ee/1 -> Product_7e168/1
  State_vq_bus_7_6865b/1 -> Product_7e168/2
  Subtract_4f174/1 -> Add_32508/1
  Product_7e168/1 -> Add_32508/2
  Add_32508/1 -> Blockout_d_iq_load_7_52844/1

== system case4/AC_1/d_iq_load_9_block ==
  note: d_iq_load_9 in case4
      | $1462.33884976487\,\mathrm{vq}_{\mathrm{bus},9}-899.932439784723\,\mathrm{iq}_{\mathrm{load},9}-376.991118430775\,\mathrm{id}_{\mathrm{load},9}$
      | Automatically generated on 2025-10-31 19:07:41 .
  State_id_load_9_3092f : Inport
  State_iq_load_9_43472 : Inport  Port=2
  State_vq_bus_9_4335e : Inport  Port=3
  Add_6aa6d : Sum
  Constant_-376.991118430775_37ddd : Constant  Value=-376.991118430775
  Constant_1462.33884976487_33d6e : Constant  Value=1462.33884976487
  Constant_899.932439784723_b7d3e : Constant  Value=899.932439784723
  Product_2ea16 : Product
  Product_406e0 : Product
  Product_c25c8 : Product
  Subtract_7ba73 : Sum  Inputs=+-
  Blockout_d_iq_load_9_a4f21 : Outport
  wires:
  Constant_-376.991118430775_37ddd/1 -> Product_406e0/1
  Product_c25c8/1 -> Subtract_7ba73/2
  State_id_load_9_3092f/1 -> Product_406e0/2
  Add_6aa6d/1 -> Blockout_d_iq_load_9_a4f21/1
  Constant_899.932439784723_b7d3e/1 -> Product_c25c8/1
  Product_2ea16/1 -> Add_6aa6d/2
  Product_406e0/1 -> Subtract_7ba73/1
  State_iq_load_9_43472/1 -> Product_c25c8/2
  Constant_1462.33884976487_33d6e/1 -> Product_2ea16/1
  State_vq_bus_9_4335e/1 -> Product_2ea16/2
  Subtract_7ba73/1 -> Add_6aa6d/1

== system case4/AC_1/d_vd_bus_1_block ==
  note: d_vd_bus_1 in case4
      | $37699111.8430775\,\mathrm{id}_{\mathrm{bus},1}+376.991118430775\,\mathrm{vq}_{\mathrm{bus},1}$
      | Automatically generated on 2025-10-31 19:07:22 .
  Alge_id_bus_1_3cc56 : Inport
  State_vq_bus_1_c46ee : Inport  Port=2
  Add_56ba6 : Sum
  Constant_376.991118430775_49e1a : Constant  Value=376.991118430775
  Constant_37699111.8430775_46de9 : Constant  Value=37699111.8430775
  Product_6ac5f : Product
  Product_e19d2 : Product
  Blockout_d_vd_bus_1_5653c : Outport
  wires:
  Constant_37699111.8430775_46de9/1 -> Product_6ac5f/1
  Product_e19d2/1 -> Add_56ba6/2
  Alge_id_bus_1_3cc56/1 -> Product_6ac5f/2
  Constant_376.991118430775_49e1a/1 -> Product_e19d2/1
  State_vq_bus_1_c46ee/1 -> Product_e19d2/2
  Add_56ba6/1 -> Blockout_d_vd_bus_1_5653c/1
  Product_6ac5f/1 -> Add_56ba6/1

== system case4/AC_1/d_vd_bus_2_block ==
  note: d_vd_bus_2 in case4
      | $37699111.8430775\,\mathrm{id}_{\mathrm{bus},2}+376.991118430775\,\mathrm{vq}_{\mathrm{bus},2}$
      | Automatically generated on 2025-10-31 19:07:23 .
  Alge_id_bus_2_da6a4 : Inport
  State_vq_bus_2_02344 : Inport  Port=2
  Add_c7071 : Sum
  Constant_376.991118430775_edddf : Constant  Value=376.991118430775
  Constant_37699111.8430775_e458f : Constant  Value=37699111.8430775
  Product_871aa : Product
  Product_e8347 : Product
  Blockout_d_vd_bus_2_d1493 : Outport
  wires:
  Constant_37699111.8430775_e458f/1 -> Product_871aa/1
  Product_e8347/1 -> Add_c7071/2
  Alge_id_bus_2_da6a4/1 -> Product_871aa/2
  Constant_376.991118430775_edddf/1 -> Product_e8347/1
  Product_871aa/1 -> Add_c7071/1
  State_vq_bus_2_02344/1 -> Product_e8347/2
  Add_c7071/1 -> Blockout_d_vd_bus_2_d1493/1

== system case4/AC_1/d_vd_bus_3_block ==
  note: d_vd_bus_3 in case4
      | $37699111.8430775\,\mathrm{id}_{\mathrm{bus},3}+376.991118430775\,\mathrm{vq}_{\mathrm{bus},3}$
      | Automatically generated on 2025-10-31 19:07:25 .
  Alge_id_bus_3_4d9b0 : Inport
  State_vq_bus_3_54d4d : Inport  Port=2
  Add_e8204 : Sum
  Constant_376.991118430775_2192f : Constant  Value=376.991118430775
  Constant_37699111.8430775_8011f : Constant  Value=37699111.8430775
  Product_6b5c7 : Product
  Product_b5c8b : Product
  Blockout_d_vd_bus_3_c41ba : Outport
  wires:
  Constant_37699111.8430775_8011f/1 -> Product_6b5c7/1
  Product_b5c8b/1 -> Add_e8204/2
  Alge_id_bus_3_4d9b0/1 -> Product_6b5c7/2
  Constant_376.991118430775_2192f/1 -> Product_b5c8b/1
  Product_6b5c7/1 -> Add_e8204/1
  State_vq_bus_3_54d4d/1 -> Product_b5c8b/2
  Add_e8204/1 -> Blockout_d_vd_bus_3_c41ba/1

== system case4/AC_1/d_vd_bus_4_block ==
  note: d_vd_bus_4 in case4
      | $2257.43184689087\,\mathrm{id}_{\mathrm{bus},4}+376.991118430775\,\mathrm{vq}_{\mathrm{bus},4}$
      | Automatically generated on 2025-10-31 19:07:27 .
  Alge_id_bus_4_12de4 : Inport
  State_vq_bus_4_d44b1 : Inport  Port=2
  Add_0ce89 : Sum
  Constant_2257.43184689087_be92b : Constant  Value=2257.43184689087
  Constant_376.991118430775_cc01c : Constant  Value=376.991118430775
  Product_c5456 : Product
  Product_ea54d : Product
  Blockout_d_vd_bus_4_acceb : Outport
  wires:
  Constant_2257.43184689087_be92b/1 -> Product_c5456/1
  Product_ea54d/1 -> Add_0ce89/2
  Alge_id_bus_4_12de4/1 -> Product_c5456/2
  Constant_376.991118430775_cc01c/1 -> Product_ea54d/1
  Product_c5456/1 -> Add_0ce89/1
  State_vq_bus_4_d44b1/1 -> Product_ea54d/2
  Add_0ce89/1 -> Blockout_d_vd_bus_4_acceb/1

== system case4/AC_1/d_vd_bus_5_block ==
  note: d_vd_bus_5 in case4
      | $1461.2058853906\,\mathrm{id}_{\mathrm{bus},5}+376.991118430775\,\mathrm{vq}_{\mathrm{bus},5}$
      | Automatically generated on 2025-10-31 19:07:28 .
  Alge_id_bus_5_5a326 : Inport
  State_vq_bus_5_bc989 : Inport  Port=2
  Add_13932 : Sum
  Constant_1461.2058853906_c3721 : Constant  Value=1461.2058853906
  Constant_376.991118430775_ccea7 : Constant  Value=376.991118430775
  Product_0a047 : Product
  Product_2109d : Product
  Blockout_d_vd_bus_5_51008 : Outport
  wires:
  Constant_1461.2058853906_c3721/1 -> Product_0a047/1
  Product_2109d/1 -> Add_13932/2
  Alge_id_bus_5_5a326/1 -> Product_0a047/2
  Constant_376.991118430775_ccea7/1 -> Product_2109d/1
  Product_0a047/1 -> Add_13932/1
  State_vq_bus_5_bc989/1 -> Product_2109d/2
  Add_13932/1 -> Blockout_d_vd_bus_5_51008/1

== system case4/AC_1/d_vd_bus_6_block ==
  note: d_vd_bus_6 in case4
      | $1329.77466818616\,\mathrm{id}_{\mathrm{bus},6}+376.991118430775\,\mathrm{vq}_{\mathrm{bus},6}$
      | Automatically generated on 2025-10-31 19:07:30 .
  Alge_id_bus_6_a9226 : Inport
  State_vq_bus_6_35b4a : Inport  Port=2
  Add_6c520 : Sum
  Constant_1329.77466818616_e4b45 : Constant  Value=1329.77466818616
  Constant_376.991118430775_4a123 : Constant  Value=376.991118430775
  Product_69511 : Product
  Product_d9eed : Product
  Blockout_d_vd_bus_6_439ef : Outport
  wires:
  Constant_1329.77466818616_e4b45/1 -> Product_69511/1
  Product_d9eed/1 -> Add_6c520/2
  Alge_id_bus_6_a9226/1 -> Product_69511/2
  Constant_376.991118430775_4a123/1 -> Product_d9eed/1
  Product_69511/1 -> Add_6c520/1
  State_vq_bus_6_35b4a/1 -> Product_d9eed/2
  Add_6c520/1 -> Blockout_d_vd_bus_6_439ef/1

== system case4/AC_1/d_vd_bus_7_block ==
  note: d_vd_bus_7 in case4
      | $2106.09563369148\,\mathrm{id}_{\mathrm{bus},7}+376.991118430775\,\mathrm{vq}_{\mathrm{bus},7}$
      | Automatically generated on 2025-10-31 19:07:31 .
  Alge_id_bus_7_14163 : Inport
  State_vq_bus_7_922d5 : Inport  Port=2
  Add_071d7 : Sum
  Constant_2106.09563369148_d25e7 : Constant  Value=2106.09563369148
  Constant_376.991118430775_69f2a : Constant  Value=376.991118430775
  Product_3903a : Product
  Product_5d403 : Product
  Blockout_d_vd_bus_7_1b5ff : Outport
  wires:
  Constant_2106.09563369148_d25e7/1 -> Product_3903a/1
  Product_5d403/1 -> Add_071d7/2
  Alge_id_bus_7_14163/1 -> Product_3903a/2
  Constant_376.991118430775_69f2a/1 -> Product_5d403/1
  Product_3903a/1 -> Add_071d7/1
  State_vq_bus_7_922d5/1 -> Product_5d403/2
  Add_071d7/1 -> Blockout_d_vd_bus_7_1b5ff/1

== system case4/AC_1/d_vd_bus_8_block ==
  note: d_vd_bus_8 in case4
      | $1657.10381727813\,\mathrm{id}_{\mathrm{bus},8}+376.991118430775\,\mathrm{vq}_{\mathrm{bus},8}$
      | Automatically generated on 2025-10-31 19:07:33 .
  Alge_id_bus_8_1a6c3 : Inport
  State_vq_bus_8_4d3d0 : Inport  Port=2
  Add_b3224 : Sum
  Constant_1657.10381727813_a2a31 : Constant  Value=1657.10381727813
  Constant_376.991118430775_91acb : Constant  Value=376.991118430775
  Product_dcb1a : Product
  Product_e5793 : Product
  Blockout_d_vd_bus_8_dd61b : Outport
  wires:
  Constant_1657.10381727813_a2a31/1 -> Product_e5793/1
  Product_dcb1a/1 -> Add_b3224/2
  Alge_id_bus_8_1a6c3/1 -> Product_e5793/2
  Constant_376.991118430775_91acb/1 -> Product_dcb1a/1
  Product_e5793/1 -> Add_b3224/1
  State_vq_bus_8_4d3d0/1 -> Product_dcb1a/2
  Add_b3224/1 -> Blockout_d_vd_bus_8_dd61b/1

== system case4/AC_1/d_vd_bus_9_block ==
  note: d_vd_bus_9 in case4
      | $1564.27849971276\,\mathrm{id}_{\mathrm{bus},9}+376.991118430775\,\mathrm{vq}_{\mathrm{bus},9}$
      | Automatically generated on 2025-10-31 19:07:34 .
  Alge_id_bus_9_57b60 : Inport
  State_vq_bus_9_f1146 : Inport  Port=2
  Add_2529d : Sum
  Constant_1564.27849971276_918f9 : Constant  Value=1564.27849971276
  Constant_376.991118430775_594cf : Constant  Value=376.991118430775
  Product_311dd : Product
  Product_dfbad : Product
  Blockout_d_vd_bus_9_6a164 : Outport
  wires:
  Constant_1564.27849971276_918f9/1 -> Product_311dd/1
  Product_dfbad/1 -> Add_2529d/2
  Alge_id_bus_9_57b60/1 -> Product_311dd/2
  Constant_376.991118430775_594cf/1 -> Product_dfbad/1
  Product_311dd/1 -> Add_2529d/1
  State_vq_bus_9_f1146/1 -> Product_dfbad/2
  Add_2529d/1 -> Blockout_d_vd_bus_9_6a164/1

== system case4/AC_1/d_vq_bus_1_block ==
  note: d_vq_bus_1 in case4
      | $37699111.8430775\,\mathrm{iq}_{\mathrm{bus},1}-376.991118430775\,\mathrm{vd}_{\mathrm{bus},1}$
      | Automatically generated on 2025-10-31 19:07:23 .
  Alge_iq_bus_1_5ed0d : Inport
  State_vd_bus_1_041f3 : Inport  Port=2
  Constant_376.991118430775_bf7a9 : Constant  Value=376.991118430775
  Constant_37699111.8430775_b8491 : Constant  Value=37699111.8430775
  Product_d4898 : Product
  Product_e7a99 : Product
  Subtract_e46d4 : Sum  Inputs=+-
  Blockout_d_vq_bus_1_40e24 : Outport
  wires:
  Constant_37699111.8430775_b8491/1 -> Product_e7a99/1
  Constant_376.991118430775_bf7a9/1 -> Product_d4898/1
  Alge_iq_bus_1_5ed0d/1 -> Product_e7a99/2
  State_vd_bus_1_041f3/1 -> Product_d4898/2
  Product_e7a99/1 -> Subtract_e46d4/1
  Product_d4898/1 -> Subtract_e46d4/2
  Subtract_e46d4/1 -> Blockout_d_vq_bus_1_40e24/1

== system case4/AC_1/d_vq_bus_2_block ==
  note: d_vq_bus_2 in case4
      | $37699111.8430775\,\mathrm{iq}_{\mathrm{bus},2}-376.991118430775\,\mathrm{vd}_{\mathrm{bus},2}$
      | Automatically generated on 2025-10-31 19:07:24 .
  Alge_iq_bus_2_66b72 : Inport
  State_vd_bus_2_c0202 : Inport  Port=2
  Constant_376.991118430775_5c222 : Constant  Value=376.991118430775
  Constant_37699111.8430775_a602c : Constant  Value=37699111.8430775
  Product_252c1 : Product
  Product_a2fd4 : Product
  Subtract_24909 : Sum  Inputs=+-
  Blockout_d_vq_bus_2_cf3a3 : Outport
  wires:
  Constant_37699111.8430775_a602c/1 -> Product_252c1/1
  Constant_376.991118430775_5c222/1 -> Product_a2fd4/1
  Alge_iq_bus_2_66b72/1 -> Product_252c1/2
  State_vd_bus_2_c0202/1 -> Product_a2fd4/2
  Product_252c1/1 -> Subtract_24909/1
  Product_a2fd4/1 -> Subtract_24909/2
  Subtract_24909/1 -> Blockout_d_vq_bus_2_cf3a3/1

== system case4/AC_1/d_vq_bus_3_block ==
  note: d_vq_bus_3 in case4
      | $37699111.8430775\,\mathrm{iq}_{\mathrm{bus},3}-376.991118430775\,\mathrm{vd}_{\mathrm{bus},3}$
      | Automatically generated on 2025-10-31 19:07:26 .
  Alge_iq_bus_3_05f49 : Inport
  State_vd_bus_3_0de91 : Inport  Port=2
  Constant_376.991118430775_ff7f9 : Constant  Value=376.991118430775
  Constant_37699111.8430775_7f44b : Constant  Value=37699111.8430775
  Product_35585 : Product
  Product_8cd9d : Product
  Subtract_9992a : Sum  Inputs=+-
  Blockout_d_vq_bus_3_13f3e : Outport
  wires:
  Constant_37699111.8430775_7f44b/1 -> Product_35585/1
  Constant_376.991118430775_ff7f9/1 -> Product_8cd9d/1
  Alge_iq_bus_3_05f49/1 -> Product_35585/2
  State_vd_bus_3_0de91/1 -> Product_8cd9d/2
  Product_35585/1 -> Subtract_9992a/1
  Product_8cd9d/1 -> Subtract_9992a/2
  Subtract_9992a/1 -> Blockout_d_vq_bus_3_13f3e/1

== system case4/AC_1/d_vq_bus_4_block ==
  note: d_vq_bus_4 in case4
      | $2257.43184689087\,\mathrm{iq}_{\mathrm{bus},4}-376.991118430775\,\mathrm{vd}_{\mathrm{bus},4}$
      | Automatically generated on 2025-10-31 19:07:27 .
  Alge_iq_bus_4_1a742 : Inport
  State_vd_bus_4_18c33 : Inport  Port=2
  Constant_2257.43184689087_10edd : Constant  Value=2257.43184689087
  Constant_376.991118430775_142b5 : Constant  Value=376.991118430775
  Product_400bd : Product
  Product_6717c : Product
  Subtract_54032 : Sum  Inputs=+-
  Blockout_d_vq_bus_4_57ae8 : Outport
  wires:
  Constant_2257.43184689087_10edd/1 -> Product_6717c/1
  Constant_376.991118430775_142b5/1 -> Product_400bd/1
  Alge_iq_bus_4_1a742/1 -> Product_6717c/2
  State_vd_bus_4_18c33/1 -> Product_400bd/2
  Product_6717c/1 -> Subtract_54032/1
  Product_400bd/1 -> Subtract_54032/2
  Subtract_54032/1 -> Blockout_d_vq_bus_4_57ae8/1

== system case4/AC_1/d_vq_bus_5_block ==
  note: d_vq_bus_5 in case4
      | $1461.2058853906\,\mathrm{iq}_{\mathrm{bus},5}-376.991118430775\,\mathrm{vd}_{\mathrm{bus},5}$
      | Automatically generated on 2025-10-31 19:07:29 .
  Alge_iq_bus_5_60a13 : Inport
  State_vd_bus_5_c20a6 : Inport  Port=2
  Constant_1461.2058853906_d0984 : Constant  Value=1461.2058853906
  Constant_376.991118430775_04eb3 : Constant  Value=376.991118430775
  Product_e0e84 : Product
  Product_e91d7 : Product
  Subtract_a5e09 : Sum  Inputs=+-
  Blockout_d_vq_bus_5_1eae7 : Outport
  wires:
  Constant_1461.2058853906_d0984/1 -> Product_e91d7/1
  Constant_376.991118430775_04eb3/1 -> Product_e0e84/1
  Alge_iq_bus_5_60a13/1 -> Product_e91d7/2
  State_vd_bus_5_c20a6/1 -> Product_e0e84/2
  Product_e91d7/1 -> Subtract_a5e09/1
  Product_e0e84/1 -> Subtract_a5e09/2
  Subtract_a5e09/1 -> Blockout_d_vq_bus_5_1eae7/1

== system case4/AC_1/d_vq_bus_6_block ==
  note: d_vq_bus_6 in case4
      | $1329.77466818616\,\mathrm{iq}_{\mathrm{bus},6}-376.991118430775\,\mathrm{vd}_{\mathrm{bus},6}$
      | Automatically generated on 2025-10-31 19:07:30 .
  Alge_iq_bus_6_7b11a : Inport
  State_vd_bus_6_cccf8 : Inport  Port=2
  Constant_1329.77466818616_a2ae6 : Constant  Value=1329.77466818616
  Constant_376.991118430775_00660 : Constant  Value=376.991118430775
  Product_00773 : Product
  Product_cfa10 : Product
  Subtract_27c8b : Sum  Inputs=+-
  Blockout_d_vq_bus_6_3e8a8 : Outport
  wires:
  Constant_1329.77466818616_a2ae6/1 -> Product_00773/1
  Constant_376.991118430775_00660/1 -> Product_cfa10/1
  Alge_iq_bus_6_7b11a/1 -> Product_00773/2
  State_vd_bus_6_cccf8/1 -> Product_cfa10/2
  Product_00773/1 -> Subtract_27c8b/1
  Product_cfa10/1 -> Subtract_27c8b/2
  Subtract_27c8b/1 -> Blockout_d_vq_bus_6_3e8a8/1
